simulink model "B5B1"  (R2015a)
settings: Solver=ode45  StartTime=0.0  StopTime=10.0  RelTol=1e-3
libraries: commfilt2 x2, dspsrcs4 x2, commchan3 x1, commsink2 x1, commutil2 x1, commanapbnd3 x1, commrandsrc2 x1, dspstat3 x1
settings Model: Creator=Ekko  LastModifiedBy=Ekko

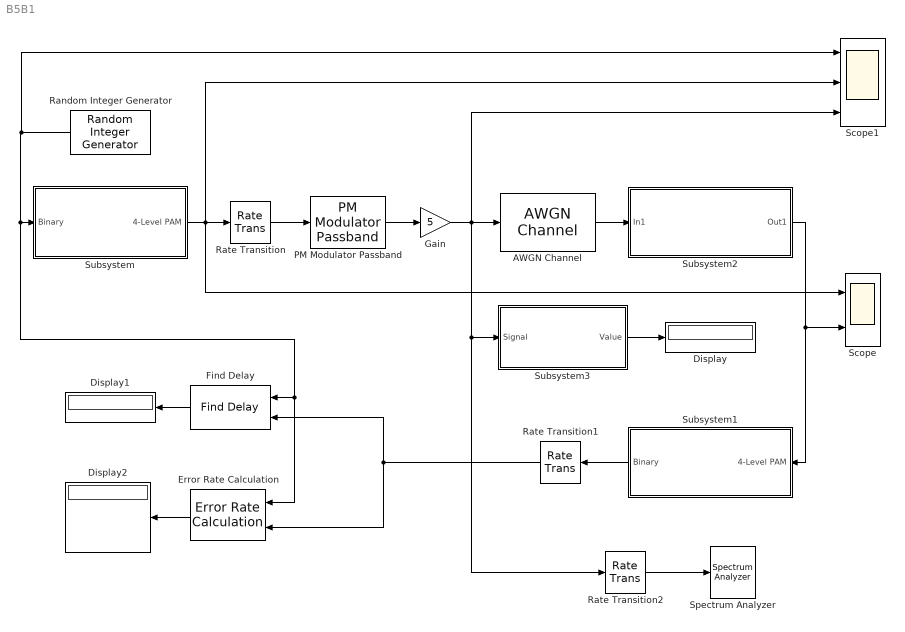
== system B5B1 ==
  AWGN Channel : commchan3/AWGN Channel  InputProcessing=Columns as channels (frame based)  seed=67  noiseMode="Signal to noise ratio  (Eb/No)"  EbNodB=12  EsNodB=10  SNRdB=10  bitsPerSym=1  Ps=1  Tsym=1  variance=1
  Display : Display
  Display1 : Display
  Display2 : Display
  Error Rate Calculation : commsink2/Error Rate Calculation  N=0  st_delay=0  cp_mode=Entire frame  subframe=[]  PMode=Port  WsName=ErrorVec  RsMode2=off  stop=off  numErr=100  maxBits=1e6
  Find Delay : commutil2/Find Delay  corrLength=200  chgSigOP=off  stopUpdate=off  numConstDelay=3
  Gain : Gain  Gain=5
  PM Modulator Passband : commanapbnd3/PM Modulator Passband  Fc=300  Ph=0  Kc=pi/2
  Random Integer Generator : commrandsrc2/Random Integer Generator  mul=2  seed=37  Ts=1e-5  frameBased=off  sampPerFrame=1  orient=off  outDataType=double
  Rate Transition : RateTransition  OutPortSampleTime=1e-5
  Rate Transition1 : RateTransition  OutPortSampleTime=1e-5
  Rate Transition2 : RateTransition  OutPortSampleTime=1e-5
  Scope : Scope  NumInputPorts=2
      settings: YMin=-5~-5  YMax=5~5
  Scope1 : Scope  NumInputPorts=3
      settings: YMin=-5~-5~-5  YMax=5~5~5
  Spectrum Analyzer : SpectrumAnalyzer
  Subsystem : Subsystem
  Subsystem1 : Subsystem
  Subsystem2 : Subsystem
  Subsystem3 : Subsystem
  wires:
  Subsystem/1(4-Level PAM) -> Scope1/2, Scope/1, Rate Transition/1
  Rate Transition/1 -> PM Modulator Passband/1
  PM Modulator Passband/1 -> Gain/1
  Gain/1 -> Rate Transition2/1, Subsystem3/1("Signal "), Scope1/3, AWGN Channel/1
  AWGN Channel/1 -> Subsystem2/1(In1)
  Subsystem1/1("Binary ") -> Rate Transition1/1
  Subsystem2/1(Out1) -> Scope/2, Subsystem1/1("4-Level PAM ")
  Random Integer Generator/1 -> Scope1/1, Find Delay/1, Error Rate Calculation/1, Subsystem/1("Binary ")
  Rate Transition2/1 -> Spectrum Analyzer/1
  Subsystem3/1("Value ") -> Display/1
  Find Delay/1 -> Display1/1
  Error Rate Calculation/1 -> Display2/1
  Rate Transition1/1 -> Error Rate Calculation/2, Find Delay/2

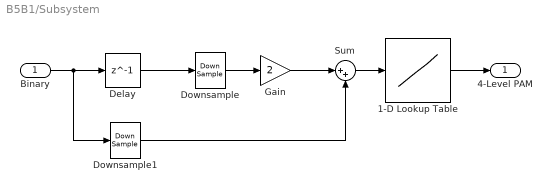
== system B5B1/Subsystem ==
  "Binary " : Inport
  1-D Lookup Table : Lookup_n-D  NumberOfTableDimensions=1  BreakpointsForDimension1=[0 1 2 3 4 5]  Table=[-5 -3 0 5 4 3]  InternalRulePriority=Speed  RndMeth=Simplest  InputSameDT=on
  Delay : Delay  DelayLength=1
  Downsample : DownSample  RateOptions=Allow multirate processing
  Downsample1 : DownSample  RateOptions=Allow multirate processing
  Gain : Gain  Gain=2
  Sum : Sum  Inputs=|++
  4-Level PAM : Outport
  wires:
  Gain/1 -> Sum/1
  Downsample1/1 -> Sum/2
  Sum/1 -> 1-D Lookup Table/1
  Delay/1 -> Downsample/1
  Downsample/1 -> Gain/1
  "Binary "/1 -> Downsample1/1, Delay/1
  1-D Lookup Table/1 -> 4-Level PAM/1

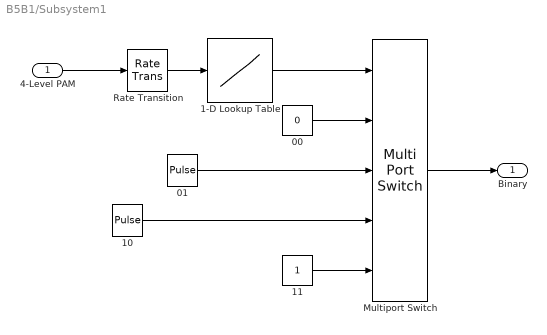
== system B5B1/Subsystem1 ==
  "4-Level PAM " : Inport
  00 : Constant  Value=0  SampleTime=2e-5
  "01 " : DiscretePulseGenerator  Amplitude=2  Period=50  PulseWidth=5  SampleTime=1e-5
  1-D Lookup Table : Lookup_n-D  NumberOfTableDimensions=1  BreakpointsForDimension1=[0 1 2 3 4 5]  Table=[-5 -3 0 5 4 3]  InternalRulePriority=Speed  RndMeth=Simplest  InputSameDT=on
  10 : DiscretePulseGenerator  Amplitude=2  Period=10  PulseWidth=5  SampleTime=1e-5
  "11 " : Constant  SampleTime=2e-5
  Multiport Switch : MultiPortSwitch  Inputs=4  DiagnosticForDefault=None
  Rate Transition : RateTransition  OutPortSampleTime=1e-5
  "Binary " : Outport
  wires:
  Rate Transition/1 -> 1-D Lookup Table/1
  "4-Level PAM "/1 -> Rate Transition/1
  1-D Lookup Table/1 -> Multiport Switch/1
  "11 "/1 -> Multiport Switch/5
  10/1 -> Multiport Switch/4
  Multiport Switch/1 -> "Binary "/1
  "01 "/1 -> Multiport Switch/3
  00/1 -> Multiport Switch/2

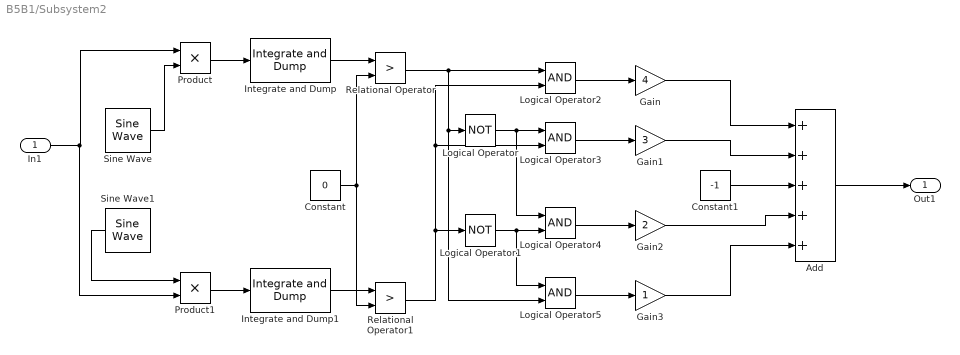
== system B5B1/Subsystem2 ==
  In1 : Inport
  Add : Sum  Inputs=5
  Constant : Constant  Value=0
  Constant1 : Constant  Value=-1
  Gain : Gain  Gain=4
  Gain1 : Gain  Gain=3
  Gain2 : Gain  Gain=2
  Gain3 : Gain
  Integrate and Dump : commfilt2/Integrate and Dump  obssamples=8  offsetsamples=0  nodump=off  roundingMode=Floor  overflowMode=off
  Integrate and Dump1 : commfilt2/Integrate and Dump  obssamples=8  offsetsamples=0  nodump=off  roundingMode=Floor  overflowMode=off
  Logical Operator : Logic  Operator=NOT  IconShape=distinctive  AllPortsSameDT=off  OutDataTypeStr=boolean
  Logical Operator1 : Logic  Operator=NOT  IconShape=distinctive  AllPortsSameDT=off  OutDataTypeStr=boolean
  Logical Operator{2..5} (4 alike) : Logic  AllPortsSameDT=off  OutDataTypeStr=boolean
  Product : Product
  Product1 : Product
  Relational Operator : RelationalOperator  Operator=>  OutDataTypeStr=boolean
  Relational Operator1 : RelationalOperator  Operator=>  OutDataTypeStr=boolean
  Sine Wave : dspsrcs4/Sine Wave  Amplitude=1  Frequency=5000  Phase=0  SampleMode=Discrete  OutComplex=Real  CompMethod=Trigonometric fcn  TableSize=Speed  SampleTime=2e-5  SamplesPerFrame=1  ResetState=Restart at time zero  dataType=double  wordLen=16  udDataType=sfix(16)  fracBitsMode=Best precision  numFracBits=15  OutDataTypeStr=double  LastOutDataTypeStr=double
  Sine Wave1 : dspsrcs4/Sine Wave  Amplitude=1  Frequency=5000  Phase=0  SampleMode=Discrete  OutComplex=Real  CompMethod=Trigonometric fcn  TableSize=Speed  SampleTime=2e-5  SamplesPerFrame=1  ResetState=Restart at time zero  dataType=double  wordLen=16  udDataType=sfix(16)  fracBitsMode=Best precision  numFracBits=15  OutDataTypeStr=double  LastOutDataTypeStr=double
  Out1 : Outport
  wires:
  In1/1 -> Product1/2, Product/1
  Integrate and Dump1/1 -> Relational Operator1/1
  Constant/1 -> Relational Operator/2, Relational Operator1/2
  Product1/1 -> Integrate and Dump1/1
  Relational Operator/1 -> Logical Operator/1, Logical Operator5/2, Logical Operator2/1
  Logical Operator4/1 -> Gain2/1
  Gain3/1 -> Add/5
  Add/1 -> Out1/1
  Logical Operator2/1 -> Gain/1
  Gain2/1 -> Add/4
  Gain1/1 -> Add/2
  Logical Operator3/1 -> Gain1/1
  Gain/1 -> Add/1
  Logical Operator5/1 -> Gain3/1
  Integrate and Dump/1 -> Relational Operator/1
  Sine Wave1/1 -> Product1/1
  Logical Operator/1 -> Logical Operator4/1, Logical Operator3/1
  Product/1 -> Integrate and Dump/1
  Constant1/1 -> Add/3
  Relational Operator1/1 -> Logical Operator1/1, Logical Operator2/2, Logical Operator3/2
  Logical Operator1/1 -> Logical Operator5/1, Logical Operator4/2
  Sine Wave/1 -> Product/2

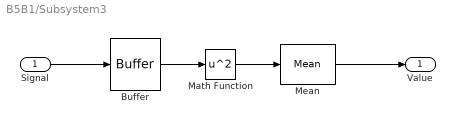
== system B5B1/Subsystem3 ==
  "Signal " : Inport
  Buffer : Buffer  TreatMby1Signals=One channel
  Math Function : Math  Operator=square  SaturateOnIntegerOverflow=on
  Mean : dspstat3/Mean  run=off  reset_popup=None  InputProcessing=Columns as channels (frame based)  directionMode=Each column  dimension=1  treatSBRowAsCol=off  roiEnable=off  roiType=Rectangles  roiPortion=Entire ROI  roiOutput=Individual statistics for each ROI  roiFlag=off  outputDataTypeStr=Inherit: Same as accumulator  outputLastDataTypeStr=Inherit: Same as accumulator  outputMin=[]  outputMax=[]  roundingMode=Floor  overflowMode=off
  "Value " : Outport
  wires:
  "Signal "/1 -> Buffer/1
  Mean/1 -> "Value "/1
  Math Function/1 -> Mean/1
  Buffer/1 -> Math Function/1
